simulink model "dspilbc"  (Simulink 8.3)
settings: Solver=FixedStepDiscrete  StartTime=0.0  StopTime=inf  RelTol=1e-3
InitFcn:
  | ilbcDatatype = get_param([bdroot '/Configuration'],'ilbcDialogDatatype');
  | if strcmp(get_param([bdroot '/Configuration'],'ilbcDialogMode'), '13.33 kbit/sec mode')
  |   ilbcMode = 1;
  | else
  |   ilbcMode = 2;
  | end
model workspace: external: MAT-File dspilbcdata.mat (data not in the file)
undefined symbols (not defined in the file or in its folder): dfilt, ilbc, Newton, Raphson
libraries: simulink x36, dspmtrx3 x27, dspsigops x13, dsparch4 x10, dspquant2 x9, dspilbclib x8, dspstat3 x8, dspsrcs4 x2, dspvision x1, dspmisc x1, dspsnks4 x1, dsplp x1
(part 1 of 3)
CloseFcn:
  | clear ilbcMode;
  | clear ilbcDatatype
settings Model: Creator=The MathWorks Inc.  ExtModeAutoUpdateStatusClock=off
settings DataIOCC: SaveOutput=off  SignalLogging=off  SaveTime=off
settings OptimizationCC: InlineParams=on  ExpressionDepthLimit=2147483647  InitFltsAndDblsToZero=on  EfficientFloat2IntCast=on  EfficientMapNaN2IntZero=off
settings DebuggingCC: InheritedTsInSrcMsg=none  SigSpecEnsureSampleTimeMsg=none  Int32ToFloatConvMsg=none  ParameterPrecisionLossMsg=none  FcnCallInpInsideContextMsg=UseLocalSettings  StrictBusMsg=ErrorOnBusTreatedAsVector
settings HardwareCC: ProdIntDivRoundTo=Floor
settings ModelReferenceCC: UpdateModelReferenceTargets=IfOutOfDate
settings SFSimCC: SimParseCustomCode=off
settings RTWCC: IncludeERTFirstTime=on
settings GRTTargetCC: TargetFcnLib=ansi_tfl_tmw_new.mat

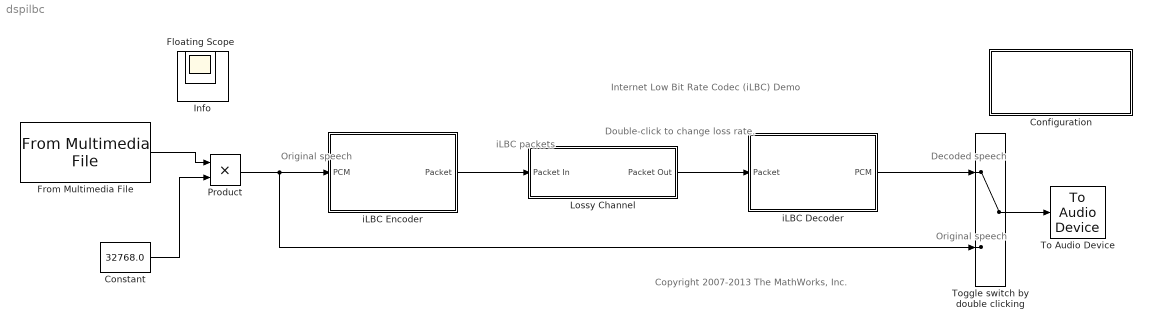
== system dspilbc ==
  note: Internet Low Bit Rate Codec (iLBC) Demo
  note: Original
      | speech
  note: iLBC
      | packets
  note: Double-click to change loss rate.
  note: Decoded
      | speech
  note: Original
      | speech
  note: Copyright 2007-2013 The MathWorks, Inc.
  Configuration : Subsystem  mask(iLBC Configuration){ilbcDialogMode=13.33 kbit/sec mode, ilbcDialogDatatype=double}
      mask prompts: ilbcDialogMode "iLBC mode:"; ilbcDialogDatatype "Internal data type:"
      mask help:
      | The iLBC standard is defined for two data rates: 13.33 kbit/sec and 15.20 kbit/sec.  Running under 13.33 kbit/sec, the encoder creates and outputs a compressed speech packet every 30ms.  With the 15.20 kbit/sec data rate, the encoder will output a packet every 20ms.  For the 13.33 kbit/sec mode, the packet size is a uint8 column vector of length 50, where each element represents one byte.  For the 15.20 kbit/sec mode, the packet is of length 38 bytes.
      |
      | The "Internal Data Type" option controls the precision for all internal floating point calculations in the iLBC Encoder and Decoder. The possible options are double and single precision.
      mask init:
      | if ilbcDialogMode == 1
      |     ilbcModeStr = '13.33';
      | elseif ilbcDialogMode == 2
      |     ilbcModeStr = '15.20';
      | end
      | 
      | if ilbcDialogDatatype == 1
      |     ilbcDatatype = 'double';
      | elseif ilbcDialogDatatype == 2
      |     ilbcDatatype = 'single';
      | end
      mask TypeOptions ilbcDialogMode: 13.33 kbit/sec mode | 15.20 kbit/sec mode
      mask TypeOptions ilbcDialogDatatype: double | single
      mask Display:
      | disp([ilbcModeStr ' kb/sec mode\n' ...
      |     'Internal data type: ' ilbcDatatype '\n' ...
      |     '[Double-click to change]']);
  Constant : Constant  Value=32768.0
  From Multimedia File : dspvision/From Multimedia File  inputFilename=speech_dft_8kHz.wav  loop=on  numPlays=inf  outputStreams=Audio only  videoDataType=single  audioDataType=double  inheritSampleTime=on  userDefinedSampleTime=1/30  noAudioOutput=off  isIntensityVideo=off  fourcc=RGB  colorVideoFormat=Separate color signals  outputEOF=off  dataOrg=Column-major  audioFrameSize=ilbc.BLOCKL{ilbcMode}  computeAudioFrameSize=off  outSamplingMode=Frame based
  Info : dspmisc/Info  SystemSampleTime=-1
  Lossy Channel : Subsystem  TreatAsAtomicUnit=on  mask(Lossy Channel){PercentLoss=3}
      mask prompts: PercentLoss "Percent of Packets Lost (0-100)"
      mask help:
      | This subsystem simulates a lossy channel by setting a specified percentage of packets to all zeros.  Enter the percentage of packets to be lost as a number in the range 0-100.
      |
      | Note that the packet loss concealment algorithm in the iLBC Decoder is tuned for packet loss rates between 0-10%.  Loss rates above 10% will result in decoded speech with clearly audible errors.
      mask Display: disp([num2str(PercentLoss) '% Random Packet Loss']);
  Product : Product  OutDataTypeStr=int16
  To Audio Device : dspsnks4/To Audio Device  deviceName=Default  inheritSampleRate=on  sampleRate=44100  deviceDatatype=Determine from input data type  autoBufferSize=on  bufferSize=4096  queueDuration=0.5  defaultOutputChannelMapping=on  outputChannelMapping=1
  Toggle switch by double clicking : ManualSwitch
  iLBC Decoder : Subsystem  TreatAsAtomicUnit=on
  iLBC Encoder : Subsystem  TreatAsAtomicUnit=on
  Floating Scope : Scope
      settings: Floating=on
  wires:
  iLBC Encoder/1(Packet) -> Lossy Channel/1(Packet In)
  Toggle switch by double clicking/1 -> To Audio Device/1
  Lossy Channel/1(Packet Out) -> iLBC Decoder/1(Packet)
  iLBC Decoder/1(PCM) -> Toggle switch by double clicking/1
  Constant/1 -> Product/2
  From Multimedia File/1 -> Product/1
  Product/1 -> Toggle switch by double clicking/2, iLBC Encoder/1(PCM)

== system dspilbc/Configuration ==

== system dspilbc/Lossy Channel ==
  Packet In : Inport
  Compare To Constant : simulink/Logic and Bit Operations/Compare To Constant  relop=>  const=PercentLoss  OutDataTypeStr=uint8  ZeroCross=off
  Gain : Gain  Gain=0  OutDataTypeStr=Inherit: Same as input
  Multiport Switch : MultiPortSwitch  DataPortOrder=Zero-based contiguous  Inputs=2  zeroidx=on
  Random Source : dspsrcs4/Random Source  SrcType=Uniform  NormMethod=Ziggurat  CltLength=12  MinVal=0  MaxVal=100  MeanVal=0  VarVal=1  RepMode=Not repeatable  rawSeed=1  IsInherit=off  SampMode=Discrete  SampTime=-1  SampFrame=1  DataType=Single  OutComplex=Real
  Packet Out : Outport
  wires:
  Multiport Switch/1 -> Packet Out/1
  Random Source/1 -> Compare To Constant/1
  Compare To Constant/1 -> Multiport Switch/1
  Packet In/1 -> Multiport Switch/3, Gain/1
  Gain/1 -> Multiport Switch/2

== system dspilbc/iLBC Decoder ==
  note: Section 4 of the iLBC standard
  Packet : Inport
  Data Type Duplicate : DataTypeDuplicate
  Data Type Duplicate1 : DataTypeDuplicate
  Data Type Conversion : DataTypeConversion  OutDataTypeStr=int16  SaturateOnIntegerOverflow=on
  Decode Sub-Blocks (4.1 - 4.4) : Subsystem
  Delay1 : dspsigops/Delay  InputProcessing=Columns as channels (frame based)  dly_unit=Frames  delay=1  ic_detail=off  dif_ic_for_ch=off  dif_ic_for_dly=off  ic=0  reset_popup=None
  Delay2 : dspsigops/Delay  InputProcessing=Columns as channels (frame based)  dly_unit=Frames  delay=1  ic_detail=off  dif_ic_for_ch=off  dif_ic_for_dly=off  ic=0  reset_popup=None
  Enable PLC : Constant  OutDataTypeStr=boolean
  High Pass Filter (4.8) : dsparch4/Digital Filter  TypePopup=IIR (poles & zeros)  IIRFiltStruct=Direct form II transposed  AllPoleFiltStruct=Direct form  FIRFiltStruct=Direct form  CoeffSource=Specify via dialog  NumCoeffs=ilbc.hpo_zero_coefsTbl  DenCoeffs=ilbc.hpo_pole_coefsTbl  BiQuadCoeffs=[1 0.3 0.4 1 0.1 0.2]  LatticeCoeffs=[0.2 0.4]  denIgnore=on  FiltPerSampPopup=One filter per frame  IC=0  ICnum=0  ICden=0  roundingMode=Floor  overflowMode=off  ScaleValues=1  scaleValueFracLength=14  stageInFracLength=15  stageOutFracLength=15  FilterSource=Specify via dialog  dfiltObjectName=dfilt.dffir([1 2 1])  InputProcessing=Columns as channels (frame based)
  Logical Operator : Logic  AllPortsSameDT=off  OutDataTypeStr=boolean
  Logical Operator1 : Logic  Operator=NOT  AllPortsSameDT=off  OutDataTypeStr=boolean
  Multiport Switch : MultiPortSwitch  DataPortOrder=Zero-based contiguous  Inputs=2  zeroidx=on
  Multiport Switch1 : MultiPortSwitch  DataPortOrder=Zero-based contiguous  Inputs=2  zeroidx=on
  Packet Loss Concealment (4.5) : Subsystem
  Saturation : Saturate  UpperLimit=32767  LowerLimit=-32768
  Set data type to back-propagate : Constant  OutDataTypeStr=ilbcDatatype
  Split Packet (3.8) : Subsystem  TreatAsAtomicUnit=on
  Synthesis Filtering (4.7) : Subsystem  TreatAsAtomicUnit=on
  PCM : Outport
  wires:
  Enable PLC/1 -> Logical Operator/2
  Set data type to back-propagate/1 -> Data Type Duplicate/1
  Logical Operator1/1 -> Logical Operator/1
  Logical Operator/1 -> Packet Loss Concealment (4.5)/Enable
  Packet Loss Concealment (4.5)/2(Synthesis) -> Multiport Switch1/2
  Packet Loss Concealment (4.5)/1(Residual) -> Multiport Switch/2
  Decode Sub-Blocks (4.1 - 4.4)/2(Synthesis) -> Data Type Duplicate1/2, Multiport Switch1/3
  Decode Sub-Blocks (4.1 - 4.4)/1(Residual) -> Multiport Switch/3
  Delay1/1 -> Packet Loss Concealment (4.5)/1(Last Residual)
  Delay2/1 -> Packet Loss Concealment (4.5)/2(Last Synthesis)
  Multiport Switch1/1 -> Data Type Duplicate1/1, Delay2/1, Synthesis Filtering (4.7)/2(Synthesis Filters)
  Multiport Switch/1 -> Delay1/1, Synthesis Filtering (4.7)/1(Residual)
  Split Packet (3.8)/8(Good Frame) -> Decode Sub-Blocks (4.1 - 4.4)/Enable, Multiport Switch1/1, Multiport Switch/1, Logical Operator1/1
  Split Packet (3.8)/1(Lsf Indices) -> Decode Sub-Blocks (4.1 - 4.4)/1(Lsf Indices)
  Split Packet (3.8)/7(Gain Indices) -> Decode Sub-Blocks (4.1 - 4.4)/7(Gain Indices)
  Split Packet (3.8)/6(Code Indices) -> Decode Sub-Blocks (4.1 - 4.4)/6(Code Indices)
  Split Packet (3.8)/5(Start State Indices) -> Decode Sub-Blocks (4.1 - 4.4)/5(Start State Indices)
  Split Packet (3.8)/4(Start State Gain Index) -> Decode Sub-Blocks (4.1 - 4.4)/4(Start State Gain Index)
  Split Packet (3.8)/3(State First) -> Decode Sub-Blocks (4.1 - 4.4)/3(State First)
  Split Packet (3.8)/2(Start State Number) -> Decode Sub-Blocks (4.1 - 4.4)/2(Start State Number)
  Synthesis Filtering (4.7)/1(Decoded Block) -> High Pass Filter (4.8)/1
  Saturation/1 -> Data Type Duplicate/2, Data Type Conversion/1
  Data Type Conversion/1 -> PCM/1
  Packet/1 -> Split Packet (3.8)/1(Packet)
  High Pass Filter (4.8)/1 -> Saturation/1

== system dspilbc/iLBC Encoder ==
  note: Section 3 of the iLBC standard
  PCM : Inport
  Calculate Residual (3.3) : Subsystem  TreatAsAtomicUnit=on
  Create Packet (3.8) : Subsystem  TreatAsAtomicUnit=on
  Data Type Conversion : DataTypeConversion  OutDataTypeStr=ilbcDatatype
  Encode Data (3.5 - 3.7) : Subsystem  TreatAsAtomicUnit=on
  Encoder LPC Analysis (3.2) : Subsystem  TreatAsAtomicUnit=on
  High Pass (3.1) : dsparch4/Digital Filter  TypePopup=IIR (poles & zeros)  IIRFiltStruct=Direct form II transposed  AllPoleFiltStruct=Direct form  FIRFiltStruct=Direct form  CoeffSource=Specify via dialog  NumCoeffs=ilbc.hpi_zero_coefsTbl  DenCoeffs=ilbc.hpi_pole_coefsTbl  BiQuadCoeffs=[1 0.3 0.4 1 0.1 0.2]  LatticeCoeffs=[0.2 0.4]  denIgnore=on  FiltPerSampPopup=One filter per frame  IC=0  ICnum=0  ICden=0  roundingMode=Floor  overflowMode=off  ScaleValues=1  scaleValueFracLength=14  stageInFracLength=15  stageOutFracLength=15  FilterSource=Specify via dialog  dfiltObjectName=dfilt.dffir([1 2 1])  InputProcessing=Columns as channels (frame based)
  Perceptual Weighting (3.4) : dspmtrx3/Array-Vector Multiply  mode=Mute  saveAsFlag=0  Dimension=1  V_Source=Dialog parameter  V_VectFromMask=ilbc.LPC_CHIRP_WEIGHTDENUM.^(0:10)'  firstCoeffSignedness=Auto  firstCoeffDataTypeStr=Inherit: Same word length as input  firstCoeffLastDataTypeStr=Inherit: Same word length as input  firstCoeffMin=[]  firstCoeffMax=[]  outputSignedness=Auto  outputDataTypeStr=Inherit: Same as product output  outputLastDataTypeStr=Inherit: Same as product output  outputMin=[]  outputMax=[]  accumSignedness=Auto  prodOutputSignedness=Auto  roundingMode=Floor  overflowMode=off
  Packet : Outport
  wires:
  Data Type Conversion/1 -> High Pass (3.1)/1
  Encoder LPC Analysis (3.2)/1(LSF Indices) -> Create Packet (3.8)/1(LSF Indices)
  High Pass (3.1)/1 -> Calculate Residual (3.3)/2(Data), Encoder LPC Analysis (3.2)/1(Data)
  Encode Data (3.5 - 3.7)/6(Gain Indices) -> Create Packet (3.8)/7(Gain Indices)
  Encode Data (3.5 - 3.7)/5(Code Indices) -> Create Packet (3.8)/6(Code Indices)
  Encode Data (3.5 - 3.7)/4(Start State Indices) -> Create Packet (3.8)/5(Start State Indices)
  Encode Data (3.5 - 3.7)/3(Start State Gain Index) -> Create Packet (3.8)/4(Start State Gain Index)
  Encode Data (3.5 - 3.7)/2(State First) -> Create Packet (3.8)/3(State First)
  Encode Data (3.5 - 3.7)/1(Start State Number) -> Create Packet (3.8)/2(Start State Number)
  Encoder LPC Analysis (3.2)/3(Weight Filters) -> Perceptual Weighting (3.4)/1
  Calculate Residual (3.3)/1(Residual) -> Encode Data (3.5 - 3.7)/3(Residual)
  Create Packet (3.8)/1(Packet) -> Packet/1
  PCM/1 -> Data Type Conversion/1
  Perceptual Weighting (3.4)/1 -> Encode Data (3.5 - 3.7)/2(Weights)
  Encoder LPC Analysis (3.2)/2(Synthesis Filters) -> Calculate Residual (3.3)/1(Synthesis Filters), Encode Data (3.5 - 3.7)/1(Synthesis)

== system dspilbc/iLBC Decoder/Decode Sub-Blocks (4.1 - 4.4) ==
  Lsf Indices : Inport
  Start State Number : Inport  Port=2
  State First : Inport  Port=3
  Start State Gain Index : Inport  Port=4
  Start State Indices : Inport  Port=5
  Code Indices : Inport  Port=6
  Gain Indices : Inport  Port=7
  Enable : EnablePort
  Decode Remaining Sub-Blocks (4.3 - 4.4) : Subsystem  TreatAsAtomicUnit=on
  Decode Start State : dspilbclib/Decode Start State
  Decoder LPC Analysis (4.1) : Subsystem  TreatAsAtomicUnit=on
  Frame Conversion2 : FrameConversion  OutFrame=Sample-based
  Selector1 : Selector  NumberOfDimensions=2  InputPortWidth=3  IndexOptions=Select all,Index vector (port)  Indices=-1,-1
  Residual : Outport
  Synthesis : Outport  Port=2
  wires:
  Frame Conversion2/1 -> Decode Remaining Sub-Blocks (4.3 - 4.4)/1(Initial Codebook)
  Start State Number/1 -> Selector1/2, Decode Remaining Sub-Blocks (4.3 - 4.4)/4(Start State Number)
  Selector1/1 -> Decode Start State/3
  State First/1 -> Decode Start State/4, Decode Remaining Sub-Blocks (4.3 - 4.4)/5(State First)
  Lsf Indices/1 -> Decoder LPC Analysis (4.1)/1(LSF Indices)
  Decoder LPC Analysis (4.1)/1(Synthesis) -> Synthesis/1, Selector1/1
  Start State Indices/1 -> Decode Start State/1
  Start State Gain Index/1 -> Decode Start State/2
  Decode Start State/1 -> Frame Conversion2/1
  Code Indices/1 -> Decode Remaining Sub-Blocks (4.3 - 4.4)/2(Code Indices)
  Gain Indices/1 -> Decode Remaining Sub-Blocks (4.3 - 4.4)/3(Gain Indices)
  Decode Remaining Sub-Blocks (4.3 - 4.4)/1(Residual) -> Residual/1

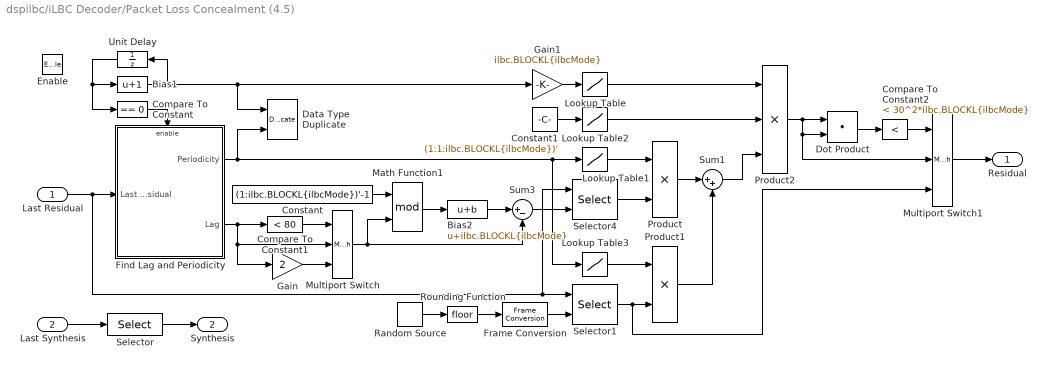
== system dspilbc/iLBC Decoder/Packet Loss Concealment (4.5) ==
  Last Residual : Inport
  Last Synthesis : Inport  Port=2
  Enable : EnablePort  StatesWhenEnabling=reset
  Bias1 : Bias  Bias=1
  Bias2 : Bias  Bias=ilbc.BLOCKL{ilbcMode}
  Compare To Constant : simulink/Logic and Bit Operations/Compare To Constant  relop===  const=0  OutDataTypeStr=boolean  ZeroCross=off
  Compare To Constant1 : simulink/Logic and Bit Operations/Compare To Constant  relop=<  const=80  OutDataTypeStr=uint8  ZeroCross=off
  Compare To Constant2 : simulink/Logic and Bit Operations/Compare To Constant  relop=<  const=30^2*ilbc.BLOCKL{ilbcMode}  OutDataTypeStr=boolean  ZeroCross=off
  Constant : Constant  Value=(1:ilbc.BLOCKL{ilbcMode})'-1  VectorParams1D=off  OutDataTypeStr=Inherit: Inherit via back propagation
  Constant1 : Constant  Value=(1:1:ilbc.BLOCKL{ilbcMode})'  VectorParams1D=off  OutDataTypeStr=Inherit: Inherit via back propagation
  Data Type Duplicate : DataTypeDuplicate
  Dot Product : DotProduct  InputSameDT=on  OutDataTypeStr=Inherit: Inherit via internal rule
  Find Lag and Periodicity : Subsystem  TreatAsAtomicUnit=on
  Frame Conversion : FrameConversion  OutFrame=Sample-based
  Gain : Gain  Gain=2  OutDataTypeStr=Inherit: Same as input
  Gain1 : Gain  Gain=ilbc.BLOCKL{ilbcMode}  OutDataTypeStr=Inherit: Inherit via back propagation  ParamDataTypeStr=Inherit: Same as input
  Lookup Table : Lookup_n-D  NumberOfTableDimensions=1  BreakpointsForDimension1=[0 320 640 960 1280]  Table=[1.0 0.9 0.7 0.5 0.0]  InterpMethod=Flat  InputSameDT=on
  Lookup Table1 : Lookup_n-D  NumberOfTableDimensions=1  BreakpointsForDimension1=[0.3 0.6]  Table=[0 1]  ExtrapMethod=Clip  InputSameDT=on
  Lookup Table2 : Lookup_n-D  NumberOfTableDimensions=1  BreakpointsForDimension1=[80 160 240]  Table=[1.00 0.95 0.90]  ExtrapMethod=Clip  InputSameDT=on
  Lookup Table3 : Lookup_n-D  NumberOfTableDimensions=1  BreakpointsForDimension1=[0.3 0.6]  Table=[1 0]  ExtrapMethod=Clip  InputSameDT=on
  Math Function1 : Math  Operator=mod  SaturateOnIntegerOverflow=on
  Multiport Switch : MultiPortSwitch  DataPortOrder=Zero-based contiguous  Inputs=2  zeroidx=on
  Multiport Switch1 : MultiPortSwitch  DataPortOrder=Zero-based contiguous  Inputs=2  zeroidx=on
  Product : Product  RndMeth=Zero
  Product1 : Product  RndMeth=Zero
  Product2 : Product  Inputs=3  RndMeth=Zero  OutDataTypeStr=Inherit: Same as first input
  Random Source : dspsrcs4/Random Source  SrcType=Uniform  NormMethod=Ziggurat  CltLength=12  MinVal=ilbc.BLOCKL{ilbcMode}-70  MaxVal=ilbc.BLOCKL{ilbcMode}-0.001  MeanVal=0  VarVal=1  RepMode=Not repeatable  rawSeed=1  IsInherit=off  SampMode=Discrete  SampTime=-1  SampFrame=ilbc.BLOCKL{ilbcMode}  DataType=Single  OutComplex=Real
  Rounding Function : Rounding
  Selector : Selector  NumberOfDimensions=2  InputPortWidth=3  IndexOptions=Select all,Index vector (dialog)  Indices=[1 3],repmat(ilbc.NSUB{ilbcMode},1,ilbc.NSUB{ilbcMode})  OutputSizes=1,1
  Selector1 : Selector  NumberOfDimensions=2  IndexMode=Zero-based  InputPortWidth=3  IndexOptions=Index vector (port),Select all  Indices=[1 3],1  OutputSizes=1,1
  Selector4 : Selector  NumberOfDimensions=2  IndexMode=Zero-based  InputPortWidth=3  IndexOptions=Index vector (port),Select all  Indices=[1 3],1  OutputSizes=1,1
  Sum1 : Sum  Inputs=|++
  Sum3 : Sum  Inputs=|+-
  Unit Delay : UnitDelay  SampleTime=-1
  Residual : Outport
  Synthesis : Outport  Port=2
  wires:
  Bias1/1 -> Data Type Duplicate/1, Gain1/1, Unit Delay/1
  Frame Conversion/1 -> Selector1/2
  Unit Delay/1 -> Compare To Constant/1, Bias1/1
  Compare To Constant/1 -> Find Lag and Periodicity/Enable
  Random Source/1 -> Rounding Function/1
  Rounding Function/1 -> Frame Conversion/1
  Gain/1 -> Multiport Switch/3
  Product1/1 -> Sum1/2
  Product/1 -> Sum1/1
  Selector1/1 -> Multiport Switch1/3, Product1/2
  Lookup Table3/1 -> Product1/1
  Selector4/1 -> Product/2
  Lookup Table1/1 -> Product/1
  Multiport Switch/1 -> Sum3/2, Math Function1/2
  Sum3/1 -> Selector4/2
  Bias2/1 -> Sum3/1
  Math Function1/1 -> Bias2/1
  Constant/1 -> Math Function1/1
  Product2/1 -> Multiport Switch1/2, Dot Product/2, Dot Product/1
  Last Residual/1 -> Selector1/1, Selector4/1, Find Lag and Periodicity/1(Last Residual)
  Lookup Table2/1 -> Product2/2
  Lookup Table/1 -> Product2/1
  Multiport Switch1/1 -> Residual/1
  Compare To Constant2/1 -> Multiport Switch1/1
  Dot Product/1 -> Compare To Constant2/1
  Sum1/1 -> Product2/3
  Constant1/1 -> Lookup Table2/1
  Gain1/1 -> Lookup Table/1
  Compare To Constant1/1 -> Multiport Switch/1
  Find Lag and Periodicity/1(Periodicity) -> Data Type Duplicate/2, Lookup Table3/1, Lookup Table1/1
  Find Lag and Periodicity/2(Lag) -> Gain/1, Multiport Switch/2, Compare To Constant1/1
  Selector/1 -> Synthesis/1
  Last Synthesis/1 -> Selector/1

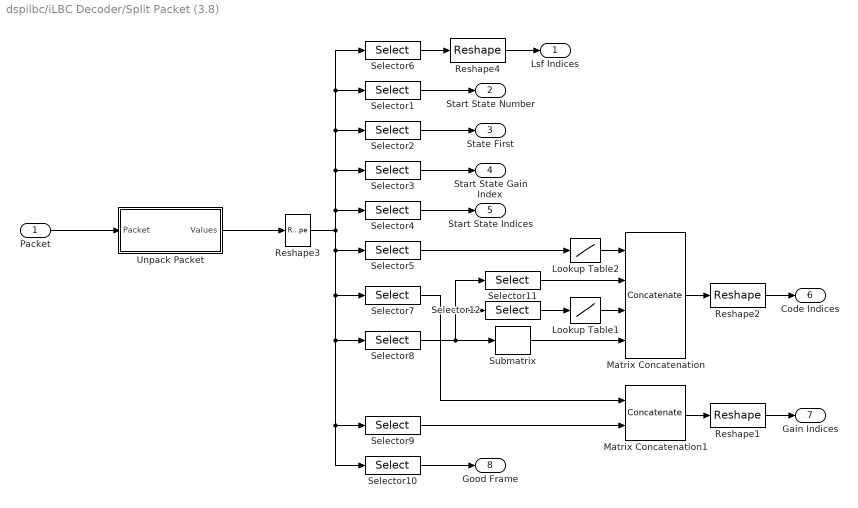
== system dspilbc/iLBC Decoder/Split Packet (3.8) ==
  Packet : Inport
  Lookup Table1 : Lookup_n-D  NumberOfTableDimensions=1  BreakpointsForDimension1=[0:255]  Table=[0:43 108:171 236:255 zeros(1,128)]  ExtrapMethod=Clip  InputSameDT=on
  Lookup Table2 : Lookup_n-D  NumberOfTableDimensions=1  BreakpointsForDimension1=[0:255]  Table=[0:57 zeros(1,6) 128:185 zeros(1,134)]  ExtrapMethod=Clip  InputSameDT=on
  Matrix Concatenation : Concatenate  NumInputs=4  Mode=Multidimensional array
  Matrix Concatenation1 : Concatenate  Mode=Multidimensional array
  Reshape1 : Reshape  OutputDimensionality=Customize  OutputDimensions=[3 (ilbc.NSUB{ilbcMode}-1)]
  Reshape2 : Reshape  OutputDimensionality=Customize  OutputDimensions=[3 (ilbc.NSUB{ilbcMode}-1)]
  Reshape3 : Reshape  OutputDimensionality=Column vector (2-D)
  Reshape4 : Reshape  OutputDimensionality=Customize  OutputDimensions=[3 (3-ilbcMode)]
  Selector1 : Selector  NumberOfDimensions=2  InputPortWidth=3  IndexOptions=Index vector (dialog),Select all  Indices=ilbc.packet_idxTbl{ilbcMode}{2},-1
  Selector10 : Selector  NumberOfDimensions=2  InputPortWidth=3  IndexOptions=Index vector (dialog),Select all  Indices=ilbc.packet_idxTbl{ilbcMode}{10},-1
  Selector11 : Selector  NumberOfDimensions=2  InputPortWidth=3  IndexOptions=Index vector (dialog),Select all  Indices=1,-1
  Selector12 : Selector  NumberOfDimensions=2  InputPortWidth=3  IndexOptions=Index vector (dialog),Select all  Indices=2:3,-1
  Selector2 : Selector  NumberOfDimensions=2  InputPortWidth=3  IndexOptions=Index vector (dialog),Select all  Indices=ilbc.packet_idxTbl{ilbcMode}{3},-1
  Selector3 : Selector  NumberOfDimensions=2  InputPortWidth=3  IndexOptions=Index vector (dialog),Select all  Indices=ilbc.packet_idxTbl{ilbcMode}{4},-1
  Selector4 : Selector  NumberOfDimensions=2  InputPortWidth=3  IndexOptions=Index vector (dialog),Select all  Indices=ilbc.packet_idxTbl{ilbcMode}{5},-1
  Selector5 : Selector  NumberOfDimensions=2  InputPortWidth=3  IndexOptions=Index vector (dialog),Select all  Indices=ilbc.packet_idxTbl{ilbcMode}{6},-1
  Selector6 : Selector  NumberOfDimensions=2  InputPortWidth=3  IndexOptions=Index vector (dialog),Select all  Indices=ilbc.packet_idxTbl{ilbcMode}{1},-1
  Selector7 : Selector  NumberOfDimensions=2  InputPortWidth=3  IndexOptions=Index vector (dialog),Select all  Indices=ilbc.packet_idxTbl{ilbcMode}{7},-1
  Selector8 : Selector  NumberOfDimensions=2  InputPortWidth=3  IndexOptions=Index vector (dialog),Select all  Indices=ilbc.packet_idxTbl{ilbcMode}{8},-1
  Selector9 : Selector  NumberOfDimensions=2  InputPortWidth=3  IndexOptions=Index vector (dialog),Select all  Indices=ilbc.packet_idxTbl{ilbcMode}{9},-1
  Submatrix : dspmtrx3/Submatrix  RowSpan=Range of rows  RowStartMode=Index  RowStartIndex=4  RowEndMode=Last  RowEndIndex=1  ColSpan=All columns  ColStartMode=First  ColStartIndex=1  ColEndMode=Last  ColEndIndex=1
  Unpack Packet : Subsystem  TreatAsAtomicUnit=on
  Lsf Indices : Outport
  Start State Number : Outport  Port=2
  State First : Outport  Port=3
  Start State Gain Index : Outport  Port=4
  Start State Indices : Outport  Port=5
  Code Indices : Outport  Port=6
  Gain Indices : Outport  Port=7
  Good Frame : Outport  Port=8
  wires:
  Unpack Packet/1(Values) -> Reshape3/1
  Packet/1 -> Unpack Packet/1(Packet)
  Lookup Table1/1 -> Matrix Concatenation/3
  Lookup Table2/1 -> Matrix Concatenation/1
  Selector12/1 -> Lookup Table1/1
  Selector11/1 -> Matrix Concatenation/2
  Submatrix/1 -> Matrix Concatenation/4
  Selector8/1 -> Submatrix/1, Selector12/1, Selector11/1
  Selector5/1 -> Lookup Table2/1
  Reshape4/1 -> Lsf Indices/1
  Reshape3/1 -> Selector1/1, Selector6/1, Selector2/1, Selector3/1, Selector4/1, Selector5/1, Selector7/1, Selector9/1, Selector10/1, Selector8/1
  Selector6/1 -> Reshape4/1
  Selector10/1 -> Good Frame/1
  Selector7/1 -> Matrix Concatenation1/1
  Selector9/1 -> Matrix Concatenation1/2
  Selector2/1 -> State First/1
  Selector4/1 -> Start State Indices/1
  Selector3/1 -> Start State Gain Index/1
  Selector1/1 -> Start State Number/1
  Reshape1/1 -> Gain Indices/1
  Reshape2/1 -> Code Indices/1
  Matrix Concatenation1/1 -> Reshape1/1
  Matrix Concatenation/1 -> Reshape2/1

== system dspilbc/iLBC Decoder/Synthesis Filtering (4.7) ==
  Residual : Inport
  Synthesis Filters : Inport  Port=2
  Assignment : Assignment  NumberOfDimensions=2  OutputInitialize=Specify size for each dimension in table  IndexOptions=Assign all,Index vector (port)  Indices=-1,1  OutputSizes=40,ilbc.NSUB{ilbcMode}
  For Iterator : ForIterator  IterationLimit=ilbc.NSUB{ilbcMode}  IterationVariableDataType=int8
  Reshape : Reshape  OutputDimensionality=Customize  OutputDimensions=[40 ilbc.NSUB{ilbcMode}]
  Reshape1 : Reshape  OutputDimensionality=Column vector (2-D)  OutputDimensions=[50 4]
  Selector1 : Selector  NumberOfDimensions=2  InputPortWidth=3  IndexOptions=Select all,Index vector (port)  Indices=-1,-1
  Selector2 : Selector  NumberOfDimensions=2  InputPortWidth=3  IndexOptions=Select all,Index vector (port)  Indices=-1,-1
  Time-Varying  Analysis Filter3 : dsparch4/Digital Filter  TypePopup=IIR (all poles)  IIRFiltStruct=Direct form II transposed  AllPoleFiltStruct=Direct form  FIRFiltStruct=Direct form  CoeffSource=Input port(s)  NumCoeffs=[1 -.95]  DenCoeffs=[1 0.1]  BiQuadCoeffs=[1 0.3 0.4 1 0.1 0.2]  LatticeCoeffs=[0.2 0.4]  denIgnore=on  FiltPerSampPopup=One filter per frame  IC=0  ICnum=0  ICden=0  roundingMode=Floor  overflowMode=off  ScaleValues=1  scaleValueFracLength=14  stageInFracLength=15  stageOutFracLength=15  FilterSource=Input port(s)  dfiltObjectName=dfilt.dffir([1 2 1])  InputProcessing=Columns as channels (frame based)
  Decoded Block : Outport
  wires:
  Reshape1/1 -> Decoded Block/1
  Assignment/1 -> Reshape1/1
  Selector1/1 -> Time-Varying  Analysis Filter3/2
  Time-Varying  Analysis Filter3/1 -> Assignment/1
  Reshape/1 -> Selector2/1
  For Iterator/1 -> Assignment/2, Selector2/2, Selector1/2
  Selector2/1 -> Time-Varying  Analysis Filter3/1
  Synthesis Filters/1 -> Selector1/1
  Residual/1 -> Reshape/1

== system dspilbc/iLBC Encoder/Calculate Residual (3.3) ==
  Synthesis Filters : Inport
  Data : Inport  Port=2
  Assignment1 : Assignment  NumberOfDimensions=2  OutputInitialize=Specify size for each dimension in table  IndexOptions=Assign all,Index vector (port)  Indices=-1,1  OutputSizes=40,ilbc.NSUB{ilbcMode}
  For Iterator : ForIterator  IterationLimit=ilbc.NSUB{ilbcMode}  IterationVariableDataType=int8
  Reshape2 : Reshape  OutputDimensionality=Customize  OutputDimensions=[40 ilbc.NSUB{ilbcMode}]
  Selector1 : Selector  NumberOfDimensions=2  InputPortWidth=3  IndexOptions=Select all,Index vector (port)  Indices=-1,-1
  Selector2 : Selector  NumberOfDimensions=2  InputPortWidth=3  IndexOptions=Select all,Index vector (port)  Indices=-1,-1
  Time-Varying  Analysis Filter1 : dsparch4/Digital Filter  TypePopup=FIR (all zeros)  IIRFiltStruct=Direct form II transposed  AllPoleFiltStruct=Direct form  FIRFiltStruct=Direct form  CoeffSource=Input port(s)  NumCoeffs=[1 -.95]  DenCoeffs=[1 0.1]  BiQuadCoeffs=[1 0.3 0.4 1 0.1 0.2]  LatticeCoeffs=[0.2 0.4]  denIgnore=on  FiltPerSampPopup=One filter per frame  IC=0  ICnum=0  ICden=0  roundingMode=Floor  overflowMode=off  ScaleValues=1  scaleValueFracLength=14  stageInFracLength=15  stageOutFracLength=15  FilterSource=Input port(s)  dfiltObjectName=dfilt.dffir([1 2 1])  InputProcessing=Columns as channels (frame based)
  Residual : Outport
  wires:
  Time-Varying  Analysis Filter1/1 -> Assignment1/1
  Selector1/1 -> Time-Varying  Analysis Filter1/2
  Selector2/1 -> Time-Varying  Analysis Filter1/1
  Assignment1/1 -> Residual/1
  Synthesis Filters/1 -> Selector1/1
  Data/1 -> Reshape2/1
  Reshape2/1 -> Selector2/1
  For Iterator/1 -> Selector1/2, Selector2/2, Assignment1/2

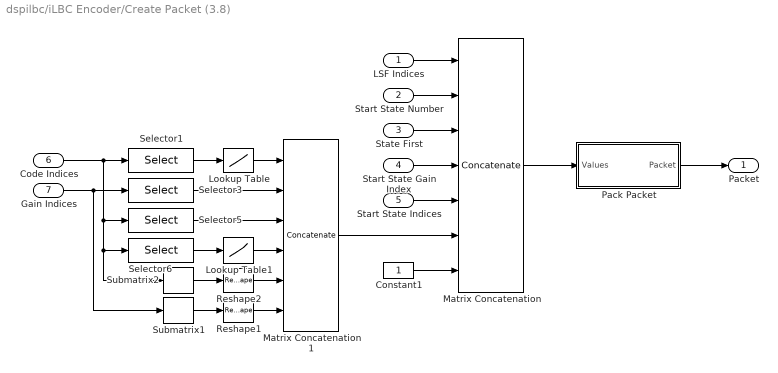
== system dspilbc/iLBC Encoder/Create Packet (3.8) ==
  LSF Indices : Inport
  Start State Number : Inport  Port=2
  State First : Inport  Port=3
  Start State Gain Index : Inport  Port=4
  Start State Indices : Inport  Port=5
  Code Indices : Inport  Port=6
  Gain Indices : Inport  Port=7
  Constant1 : Constant  OutDataTypeStr=uint8
  Lookup Table : Lookup_n-D  NumberOfTableDimensions=1  BreakpointsForDimension1=[0:255]  Table=[0:57 zeros(1,70) 64:121 zeros(1,70)]  ExtrapMethod=Clip  InputSameDT=on
  Lookup Table1 : Lookup_n-D  NumberOfTableDimensions=1  BreakpointsForDimension1=[0:255]  Table=[0:43 zeros(1,64) 44:107 zeros(1,64) 108:127]  ExtrapMethod=Clip  InputSameDT=on
  Matrix Concatenation : Concatenate  NumInputs=7  Mode=Multidimensional array
  Matrix Concatenation1 : Concatenate  NumInputs=6  Mode=Multidimensional array
  Pack Packet : Subsystem  TreatAsAtomicUnit=on
  Reshape1 : Reshape  OutputDimensionality=Column vector (2-D)
  Reshape2 : Reshape  OutputDimensionality=Column vector (2-D)
  Selector1 : Selector  NumberOfDimensions=2  InputPortWidth=3  IndexOptions=Select all,Index vector (dialog)  Indices=-1,1
  Selector3 : Selector  NumberOfDimensions=2  InputPortWidth=3  IndexOptions=Select all,Index vector (dialog)  Indices=-1,1
  Selector5 : Selector  NumberOfDimensions=2  InputPortWidth=3  IndexOptions=Index vector (dialog),Index vector (dialog)  Indices=1,2
  Selector6 : Selector  NumberOfDimensions=2  InputPortWidth=3  IndexOptions=Index vector (dialog),Index vector (dialog)  Indices=2:3,2
  Submatrix1 : dspmtrx3/Submatrix  RowSpan=All rows  RowStartMode=First  RowStartIndex=1  RowEndMode=Last  RowEndIndex=1  ColSpan=Range of columns  ColStartMode=Index  ColStartIndex=2  ColEndMode=Last  ColEndIndex=1
  Submatrix2 : dspmtrx3/Submatrix  RowSpan=All rows  RowStartMode=First  RowStartIndex=1  RowEndMode=Last  RowEndIndex=1  ColSpan=Range of columns  ColStartMode=Index  ColStartIndex=3  ColEndMode=Last  ColEndIndex=1
  Packet : Outport
  wires:
  Pack Packet/1(Packet) -> Packet/1
  Matrix Concatenation/1 -> Pack Packet/1(Values)
  Lookup Table1/1 -> Matrix Concatenation1/4
  Lookup Table/1 -> Matrix Concatenation1/1
  Selector3/1 -> Matrix Concatenation1/2
  Gain Indices/1 -> Submatrix1/1, Selector3/1
  Reshape1/1 -> Matrix Concatenation1/6
  Reshape2/1 -> Matrix Concatenation1/5
  Submatrix2/1 -> Reshape2/1
  Selector5/1 -> Matrix Concatenation1/3
  Selector6/1 -> Lookup Table1/1
  Submatrix1/1 -> Reshape1/1
  Matrix Concatenation1/1 -> Matrix Concatenation/6
  Selector1/1 -> Lookup Table/1
  Code Indices/1 -> Submatrix2/1, Selector6/1, Selector5/1, Selector1/1
  Constant1/1 -> Matrix Concatenation/7
  Start State Indices/1 -> Matrix Concatenation/5
  Start State Gain Index/1 -> Matrix Concatenation/4
  State First/1 -> Matrix Concatenation/3
  Start State Number/1 -> Matrix Concatenation/2
  LSF Indices/1 -> Matrix Concatenation/1

== system dspilbc/iLBC Encoder/Encode Data (3.5 - 3.7) ==
  Synthesis : Inport
  Weights : Inport  Port=2
  Residual : Inport  Port=3
  Decode Start State (3.5.3 last paragraph) : dspilbclib/Decode Start State
  Encode Remaining Sub-Blocks (3.6 - 3.7) : Subsystem
  Encode Start State (3.5.2 - 3.5.3) : Subsystem  TreatAsAtomicUnit=on
  Extract Sub-Blocks (3.5.1) and Sort LPC Filters : Subsystem  TreatAsAtomicUnit=on
  Start State Number : Outport
  State First : Outport  Port=2
  Start State Gain Index : Outport  Port=3
  Start State Indices : Outport  Port=4
  Code Indices : Outport  Port=5
  Gain Indices : Outport  Port=6
  wires:
  Extract Sub-Blocks (3.5.1) and Sort LPC Filters/3(Start State Number) -> Start State Number/1, Encode Remaining Sub-Blocks (3.6 - 3.7)/3(Start State Number)
  Extract Sub-Blocks (3.5.1) and Sort LPC Filters/7(Start State Synthesis) -> Decode Start State (3.5.3 last paragraph)/3, Encode Start State (3.5.2 - 3.5.3)/3(Synthesis Filter)
  Extract Sub-Blocks (3.5.1) and Sort LPC Filters/6(Start State Weights) -> Encode Start State (3.5.2 - 3.5.3)/2(Weight Filters)
  Extract Sub-Blocks (3.5.1) and Sort LPC Filters/5(Start State) -> Encode Start State (3.5.2 - 3.5.3)/1(Start State)
  Weights/1 -> Extract Sub-Blocks (3.5.1) and Sort LPC Filters/3(Weights)
  Extract Sub-Blocks (3.5.1) and Sort LPC Filters/2(Sorted Weights) -> Encode Remaining Sub-Blocks (3.6 - 3.7)/2(Weights)
  Extract Sub-Blocks (3.5.1) and Sort LPC Filters/1(Sorted Sub-blocks) -> Encode Remaining Sub-Blocks (3.6 - 3.7)/1(Sub-blocks)
  Synthesis/1 -> Extract Sub-Blocks (3.5.1) and Sort LPC Filters/2(Synthesis)
  Encode Start State (3.5.2 - 3.5.3)/2(Start State Gain Index) -> Start State Gain Index/1, Decode Start State (3.5.3 last paragraph)/2
  Decode Start State (3.5.3 last paragraph)/1 -> Encode Remaining Sub-Blocks (3.6 - 3.7)/5(Initial Codebook)
  Encode Remaining Sub-Blocks (3.6 - 3.7)/2(Gains) -> Gain Indices/1
  Encode Remaining Sub-Blocks (3.6 - 3.7)/1(Codes) -> Code Indices/1
  Encode Start State (3.5.2 - 3.5.3)/1(Start State Indices) -> Start State Indices/1, Decode Start State (3.5.3 last paragraph)/1
  Residual/1 -> Extract Sub-Blocks (3.5.1) and Sort LPC Filters/1(Residual)
  Extract Sub-Blocks (3.5.1) and Sort LPC Filters/4(State First) -> Encode Remaining Sub-Blocks (3.6 - 3.7)/4(State First), State First/1, Decode Start State (3.5.3 last paragraph)/4, Encode Start State (3.5.2 - 3.5.3)/4(State First)

== system dspilbc/iLBC Encoder/Encoder LPC Analysis (3.2) ==
  note: 3.2.1
  note: 3.2.2
  note: 3.2.3
  Data : Inport
  Autocorrelation : dspstat3/Autocorrelation  AllPositiveLags=off  maxlag=10  bias=None  domain=Time  outputDataTypeStr=Inherit: Same as accumulator  outputLastDataTypeStr=Inherit: Same as accumulator  outputMin=[]  outputMax=[]  roundingMode=Floor  overflowMode=off
  Delay2 : dspsigops/Delay  InputProcessing=Columns as channels (frame based)  dly_unit=Frames  delay=1  ic_detail=off  dif_ic_for_ch=off  dif_ic_for_dly=off  ic=0  reset_popup=None
  Find Perceptual Weight Filters (3.2.6) : dspilbclib/Find LPC Filters
  Find Synthesis Filters (3.2.6) : dspilbclib/Find LPC Filters
  Frame Conversion1 : FrameConversion
  Gain : Gain  Gain=ilbc.lpc_winTbls{ilbcMode}
  LPC to LSF/LSP Conversion1 : dsplp/LPC to LSF//LSP Conversion  output=LSF in range (0 pi)  NSteps=64  NBisects=6  RootStatus=off  correction=off  lastLSP=off  error=Ignore
  LSF Quantization (3.2.4) : Subsystem
  Levinson-Durbin : dspsolvers/Levinson-Durbin  coeffOutFcn=OBSOLETE  coeffOutFcnActive=A  outP=off  zeroInpHandling=on  firstCoeffMode=Binary point scaling  firstCoeffWordLength=16  firstCoeffFracLength=15  firstCoeffDataTypeStr=fixdt(1,16,15)  firstCoeffLastDataTypeStr=fixdt(1,16,15)  firstCoeffMin=[]  firstCoeffMax=[]  secondCoeffMode=Binary point scaling  secondCoeffWordLength=16  secondCoeffFracLength=15  secondCoeffDataTypeStr=fixdt(1,16,15)  secondCoeffLastDataTypeStr=fixdt(1,16,15)  secondCoeffMin=[]  secondCoeffMax=[]  outputMin=[]  outputMax=[]  accumMode=Binary point scaling  accumWordLength=32  accumFracLength=30  accumDataTypeStr=fixdt(1,32,30)  accumLastDataTypeStr=fixdt(1,32,30)  prodOutputMode=Binary point scaling  prodOutputWordLength=32  prodOutputFracLength=30  prodOutputDataTypeStr=fixdt(1,32,30)  prodOutputLastDataTypeStr=fixdt(1,32,30)  roundingMode=Floor  overflowMode=off
      settings: allowOverrides=off
  Matrix Concatenation3 : Concatenate  Mode=Multidimensional array
  Matrix Scaling : dspmtrx3/Array-Vector Multiply  mode=Mute  saveAsFlag=0  Dimension=1  V_Source=Dialog parameter  V_VectFromMask=ilbc.lpc_lagwinTbl  firstCoeffSignedness=Auto  firstCoeffDataTypeStr=Inherit: Same word length as input  firstCoeffLastDataTypeStr=Inherit: Same word length as input  firstCoeffMin=[]  firstCoeffMax=[]  outputSignedness=Auto  outputDataTypeStr=Inherit: Same as product output  outputLastDataTypeStr=Inherit: Same as product output  outputMin=[]  outputMax=[]  accumSignedness=Auto  prodOutputSignedness=Auto  roundingMode=Floor  overflowMode=off
  Matrix Scaling1 : dspmtrx3/Array-Vector Multiply  mode=Mute  saveAsFlag=0  Dimension=1  V_Source=Dialog parameter  V_VectFromMask=ilbc.LPC_CHIRP_SYNTDENUM.^(0:10)'  firstCoeffSignedness=Auto  firstCoeffDataTypeStr=Inherit: Same word length as input  firstCoeffLastDataTypeStr=Inherit: Same word length as input  firstCoeffMin=[]  firstCoeffMax=[]  outputSignedness=Auto  outputDataTypeStr=Inherit: Same as product output  outputLastDataTypeStr=Inherit: Same as product output  outputMin=[]  outputMax=[]  accumSignedness=Auto  prodOutputSignedness=Auto  roundingMode=Floor  overflowMode=off
  Reshape : Reshape  OutputDimensionality=Customize  OutputDimensions=[240 (3-ilbcMode)]
  Selector : Selector  NumberOfDimensions=2  InputPortWidth=3  IndexOptions=Index vector (dialog),Index vector (dialog)  Indices=ilbc.lpc_winIdxTbl{ilbcMode},1  OutputSizes=1,1
  Submatrix1 : dspmtrx3/Submatrix  RowSpan=Range of rows  RowStartMode=Offset from last  RowStartIndex=ilbc.BUFFEROVERLAP{ilbcMode}-1  RowEndMode=Last  RowEndIndex=1  ColSpan=All columns  ColStartMode=Offset from last  ColStartIndex=1  ColEndMode=Last  ColEndIndex=1
  LSF Indices : Outport
  Synthesis Filters : Outport  Port=2
  Weight Filters : Outport  Port=3
  wires:
  Matrix Concatenation3/1 -> Selector/1
  Data/1 -> Matrix Concatenation3/2, Submatrix1/1
  Submatrix1/1 -> Delay2/1
  Delay2/1 -> Matrix Concatenation3/1
  Selector/1 -> Reshape/1
  Autocorrelation/1 -> Matrix Scaling/1
  LSF Quantization (3.2.4)/2(Quantized LSF Vectors) -> Find Synthesis Filters (3.2.6)/1
  Gain/1 -> Autocorrelation/1
  LSF Quantization (3.2.4)/1(LSF Indices) -> LSF Indices/1
  Reshape/1 -> Gain/1
  Levinson-Durbin/1 -> Matrix Scaling1/1
  Matrix Scaling1/1 -> LPC to LSF/LSP Conversion1/1
  Find Synthesis Filters (3.2.6)/1 -> Synthesis Filters/1
  Find Perceptual Weight Filters (3.2.6)/1 -> Weight Filters/1
  Frame Conversion1/1 -> LSF Quantization (3.2.4)/1(LSF Vectors), Find Perceptual Weight Filters (3.2.6)/1
  LPC to LSF/LSP Conversion1/1 -> Frame Conversion1/1
  Matrix Scaling/1 -> Levinson-Durbin/1

== system dspilbc/iLBC Decoder/Decode Sub-Blocks (4.1 - 4.4)/Decode Remaining Sub-Blocks (4.3 - 4.4) ==
  Initial Codebook : Inport
  Code Indices : Inport  Port=2
  Gain Indices : Inport  Port=3
  Start State Number : Inport  Port=4
  State First : Inport  Port=5
  Compare To Constant2 : simulink/Logic and Bit Operations/Compare To Constant  relop=>  const=0  OutDataTypeStr=uint8  ZeroCross=off
  Decode Remaining Sub-Blocks (4.3 - 4.4) : dspilbclib/Decode Sub-Block
  For Iterator : ForIterator  ResetStates=reset  IterationLimit=ilbc.NSUB{ilbcMode}-1  IndexMode=Zero-based
  Frame Conversion1 : FrameConversion  OutFrame=Sample-based
  Frame Conversion3 : FrameConversion
  Pad : dspsigops/Pad  padAlong=Columns  dimsToPad=1  valSrc=Specify via dialog  padVal=0  spec=Pad size  padNumOutRowsSpecMethod=User-specified  numOutRows=ilbc.BLOCKL{ilbcMode}-40  padNumOutColsSpecMethod=User-specified  numOutCols=1  isVarDimsMode=off  padBeginning=90  padEnd=0  outSizeMode=User-specified  outSize=1  padSigAt=Beginning  trunc_flag=None  roundingMode=Floor  overflowMode=off  truncOrWrapMode=Truncate  wrap_flag=None
  Selector1 : Selector  NumberOfDimensions=2  IndexMode=Zero-based  InputPortWidth=3  IndexOptions=Select all,Index vector (port)  Indices=-1,0
  Selector3 : Selector  NumberOfDimensions=2  IndexMode=Zero-based  InputPortWidth=3  IndexOptions=Select all,Index vector (port)  Indices=-1,0
  Submatrix : dspmtrx3/Submatrix  RowSpan=Range of rows  RowStartMode=Index  RowStartIndex=41  RowEndMode=Last  RowEndIndex=1  ColSpan=All columns  ColStartMode=First  ColStartIndex=1  ColEndMode=Last  ColEndIndex=1
  Unit Delay External IC : simulink/Additional Math & Discrete/Additional Discrete/Unit Delay External IC  tsamp=-1
  Residual : Outport
  wires:
  For Iterator/1 -> Selector3/2, Compare To Constant2/1, Selector1/2, Decode Remaining Sub-Blocks (4.3 - 4.4)/5
  Frame Conversion1/1 -> Submatrix/1
  Selector3/1 -> Decode Remaining Sub-Blocks (4.3 - 4.4)/3
  Selector1/1 -> Decode Remaining Sub-Blocks (4.3 - 4.4)/4
  Unit Delay External IC/1 -> Frame Conversion3/1
  Gain Indices/1 -> Selector1/1
  Code Indices/1 -> Selector3/1
  Initial Codebook/1 -> Pad/1
  Decode Remaining Sub-Blocks (4.3 - 4.4)/1 -> Residual/1, Frame Conversion1/1
  Submatrix/1 -> Unit Delay External IC/1
  Pad/1 -> Unit Delay External IC/2
  Frame Conversion3/1 -> Decode Remaining Sub-Blocks (4.3 - 4.4)/1
  Compare To Constant2/1 -> Decode Remaining Sub-Blocks (4.3 - 4.4)/2
  Start State Number/1 -> Decode Remaining Sub-Blocks (4.3 - 4.4)/6
  State First/1 -> Decode Remaining Sub-Blocks (4.3 - 4.4)/7

== system dspilbc/iLBC Decoder/Decode Sub-Blocks (4.1 - 4.4)/Decoder LPC Analysis (4.1) ==
  LSF Indices : Inport
  Concatenation of Quantized LSFs : Concatenate  NumInputs=3  Mode=Multidimensional array
  Find Synthesis Filters (3.2.6) : dspilbclib/Find LPC Filters
  Frame Conversion1 : FrameConversion
  Selector3 : Selector  NumberOfDimensions=2  InputPortWidth=3  IndexOptions=Index vector (dialog),Select all  Indices=1,-1
  Selector4 : Selector  NumberOfDimensions=2  InputPortWidth=3  IndexOptions=Index vector (dialog),Select all  Indices=2,-1
  Selector5 : Selector  NumberOfDimensions=2  InputPortWidth=3  IndexOptions=Index vector (dialog),Select all  Indices=3,-1
  Sort : dspstat3/Sort  otype=Value  dir=Ascending  sortAlg=Quick sort  roundingMode=Floor  overflowMode=off
  Vector Quantizer Decoder1 : dspquant2/Vector Quantizer Decoder  invalidin=Clip  CBsource=Specify via dialog  codebook=ilbc.lsfCbTbl1  dataType=Inherit via back propagation  isSigned=on  wordLen=16  udDataType=float('single')  fracBitsMode=Best precision  numFracBits=7  OutDataTypeStr=Inherit: Inherit via back propagation  LastOutDataTypeStr=Inherit: Inherit via back propagation
  Vector Quantizer Decoder2 : dspquant2/Vector Quantizer Decoder  invalidin=Clip  CBsource=Specify via dialog  codebook=ilbc.lsfCbTbl2  dataType=Inherit via back propagation  isSigned=on  wordLen=16  udDataType=float('single')  fracBitsMode=Best precision  numFracBits=7  OutDataTypeStr=Inherit: Inherit via back propagation  LastOutDataTypeStr=Inherit: Inherit via back propagation
  Vector Quantizer Decoder3 : dspquant2/Vector Quantizer Decoder  invalidin=Clip  CBsource=Specify via dialog  codebook=ilbc.lsfCbTbl3  dataType=Inherit via back propagation  isSigned=on  wordLen=16  udDataType=float('single')  fracBitsMode=Best precision  numFracBits=7  OutDataTypeStr=Inherit: Inherit via back propagation  LastOutDataTypeStr=Inherit: Inherit via back propagation
  Synthesis : Outport
  wires:
  Frame Conversion1/1 -> Selector3/1, Selector4/1, Selector5/1
  Find Synthesis Filters (3.2.6)/1 -> Synthesis/1
  Sort/1 -> Find Synthesis Filters (3.2.6)/1
  Concatenation of Quantized LSFs/1 -> Sort/1
  Vector Quantizer Decoder3/1 -> Concatenation of Quantized LSFs/3
  Vector Quantizer Decoder2/1 -> Concatenation of Quantized LSFs/2
  Vector Quantizer Decoder1/1 -> Concatenation of Quantized LSFs/1
  LSF Indices/1 -> Frame Conversion1/1
  Selector5/1 -> Vector Quantizer Decoder3/1
  Selector4/1 -> Vector Quantizer Decoder2/1
  Selector3/1 -> Vector Quantizer Decoder1/1

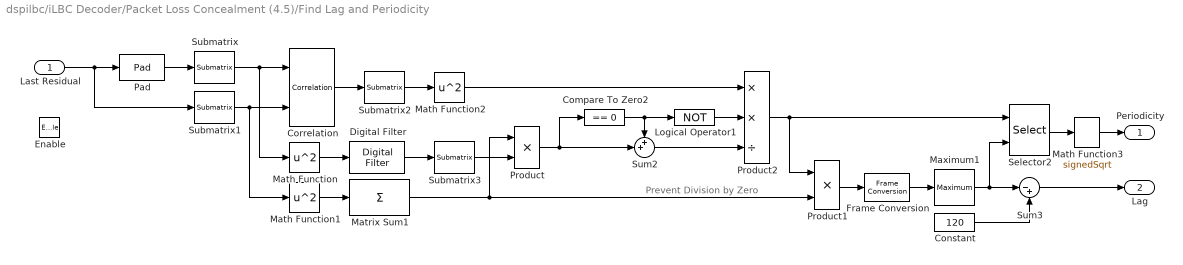
== system dspilbc/iLBC Decoder/Packet Loss Concealment (4.5)/Find Lag and Periodicity ==
  note: Prevent Division by Zero
  Last Residual : Inport
  Enable : EnablePort
  Compare To Zero2 : simulink/Logic and Bit Operations/Compare To Zero  relop===  OutDataTypeStr=uint8  ZeroCross=off
  Constant : Constant  Value=120  OutDataTypeStr=Inherit: Inherit via back propagation
  Correlation : dspstat3/Correlation  domain=Time  outputDataTypeStr=Inherit: Same as accumulator  outputLastDataTypeStr=Inherit: Same as accumulator  outputMin=[]  outputMax=[]  roundingMode=Floor  overflowMode=off
  Digital Filter : dsparch4/Digital Filter  TypePopup=FIR (all zeros)  IIRFiltStruct=Direct form II transposed  AllPoleFiltStruct=Direct form  FIRFiltStruct=Direct form  CoeffSource=Specify via dialog  NumCoeffs=ones(60,1)  DenCoeffs=[1 0.1]  BiQuadCoeffs=[1 0.3 0.4 1 0.1 0.2]  LatticeCoeffs=[0.2 0.4]  denIgnore=on  FiltPerSampPopup=One filter per frame  IC=0  ICnum=0  ICden=0  roundingMode=Floor  overflowMode=off  ScaleValues=1  scaleValueFracLength=14  stageInFracLength=15  stageOutFracLength=15  FilterSource=Specify via dialog  dfiltObjectName=dfilt.dffir([1 2 1])  InputProcessing=Columns as channels (frame based)
  Frame Conversion : FrameConversion  OutFrame=Sample-based
  Logical Operator1 : Logic  Operator=NOT  AllPortsSameDT=off  OutDataTypeStr=boolean
  Math Function : Math  Operator=square  SaturateOnIntegerOverflow=on
  Math Function1 : Math  Operator=square  SaturateOnIntegerOverflow=on
  Math Function2 : Math  Operator=square  SaturateOnIntegerOverflow=on
  Math Function3 : Sqrt  Operator=signedSqrt  AlgorithmType=Newton-Raphson  SaturateOnIntegerOverflow=on
  Matrix Sum1 : Sum  Inputs=+  CollapseMode=Specified dimension  OutDataTypeStr=Inherit: Same as accumulator
  Maximum1 : dspstat3/Maximum  fcn=Index  reset=None  InputProcessing=Columns as channels (frame based)  indexBase=Zero  operateOver=Each column  Dimension=1  colComp=on  operation=maximum  roiEnable=off  roiType=Rectangles  roiPortion=Entire ROI  roiOutput=Individual statistics for each ROI  roiFlag=off  accumDataTypeStr=Inherit: Same as product output  accumLastDataTypeStr=Inherit: Same as product output  roundingMode=Floor  overflowMode=off
  Pad : dspsigops/Pad  padAlong=Columns  dimsToPad=1  valSrc=Specify via dialog  padVal=0  spec=Output size  padNumOutRowsSpecMethod=User-specified  numOutRows=60+120  padNumOutColsSpecMethod=User-specified  numOutCols=1  isVarDimsMode=off  padBeginning=0  padEnd=0  outSizeMode=User-specified  outSize=1  padSigAt=Beginning  trunc_flag=None  roundingMode=Floor  overflowMode=off  truncOrWrapMode=Truncate  wrap_flag=None
  Product : Product  RndMeth=Zero
  Product1 : Product  RndMeth=Zero
  Product2 : Product  Inputs=**/  RndMeth=Zero
  Selector2 : Selector  NumberOfDimensions=2  IndexMode=Zero-based  InputPortWidth=3  IndexOptions=Index vector (port),Index vector (dialog)  Indices=[1 3],0  OutputSizes=7,1
  Submatrix : dspmtrx3/Submatrix  RowSpan=Range of rows  RowStartMode=First  RowStartIndex=120+60-1  RowEndMode=Offset from last  RowEndIndex=20  ColSpan=All columns  ColStartMode=First  ColStartIndex=1  ColEndMode=Last  ColEndIndex=1
  Submatrix1 : dspmtrx3/Submatrix  RowSpan=Range of rows  RowStartMode=Offset from last  RowStartIndex=60-1  RowEndMode=Last  RowEndIndex=60  ColSpan=All columns  ColStartMode=First  ColStartIndex=1  ColEndMode=Last  ColEndIndex=1
  Submatrix2 : dspmtrx3/Submatrix  RowSpan=Range of rows  RowStartMode=Index  RowStartIndex=60  RowEndMode=Offset from last  RowEndIndex=60-1  ColSpan=All columns  ColStartMode=First  ColStartIndex=1  ColEndMode=Last  ColEndIndex=1
  Submatrix3 : dspmtrx3/Submatrix  RowSpan=Range of rows  RowStartMode=Offset from last  RowStartIndex=100  RowEndMode=Last  RowEndIndex=101  ColSpan=All columns  ColStartMode=First  ColStartIndex=1  ColEndMode=Last  ColEndIndex=1
  Sum2 : Sum  Inputs=++|
  Sum3 : Sum  Inputs=|-+
  Periodicity : Outport
  Lag : Outport  Port=2
  wires:
  Compare To Zero2/1 -> Sum2/1, Logical Operator1/1
  Logical Operator1/1 -> Product2/2
  Submatrix3/1 -> Product/2
  Math Function3/1 -> Periodicity/1
  Constant/1 -> Sum3/2
  Frame Conversion/1 -> Maximum1/1
  Math Function2/1 -> Product2/1
  Maximum1/1 -> Sum3/1, Selector2/2
  Submatrix/1 -> Correlation/1, Math Function/1
  Submatrix1/1 -> Math Function1/1, Correlation/2
  Sum3/1 -> Lag/1
  Selector2/1 -> Math Function3/1
  Product2/1 -> Selector2/1, Product1/1
  Product1/1 -> Frame Conversion/1
  Sum2/1 -> Product2/3
  Product/1 -> Compare To Zero2/1, Sum2/2
  Matrix Sum1/1 -> Product/1, Product1/2
  Digital Filter/1 -> Submatrix3/1
  Math Function/1 -> Digital Filter/1
  Math Function1/1 -> Matrix Sum1/1
  Pad/1 -> Submatrix/1
  Submatrix2/1 -> Math Function2/1
  Correlation/1 -> Submatrix2/1
  Last Residual/1 -> Submatrix1/1, Pad/1

== system dspilbc/iLBC Decoder/Split Packet (3.8)/Unpack Packet ==
  Packet : Inport
  Assignment : Assignment  Indices=ilbc.bit_packTbl{ilbcMode}
  Bitwise Operator1 : simulink/Logic and Bit Operations/Bitwise Operator  logicop=AND  UseBitMask=on  BitMask=128  BitMaskRealWorld=Stored Integer
  Bitwise Operator2 : simulink/Logic and Bit Operations/Bitwise Operator  logicop=AND  UseBitMask=on  BitMask=64  BitMaskRealWorld=Stored Integer
  Bitwise Operator3 : simulink/Logic and Bit Operations/Bitwise Operator  logicop=AND  UseBitMask=on  BitMask=32  BitMaskRealWorld=Stored Integer
  Bitwise Operator4 : simulink/Logic and Bit Operations/Bitwise Operator  logicop=AND  UseBitMask=on  BitMask=16  BitMaskRealWorld=Stored Integer
  Bitwise Operator5 : simulink/Logic and Bit Operations/Bitwise Operator  logicop=AND  UseBitMask=on  BitMask=8  BitMaskRealWorld=Stored Integer
  Bitwise Operator6 : simulink/Logic and Bit Operations/Bitwise Operator  logicop=AND  UseBitMask=on  BitMask=4  BitMaskRealWorld=Stored Integer
  Bitwise Operator7 : simulink/Logic and Bit Operations/Bitwise Operator  logicop=AND  UseBitMask=on  BitMask=2  BitMaskRealWorld=Stored Integer
  Bitwise Operator8 : simulink/Logic and Bit Operations/Bitwise Operator  logicop=AND  UseBitMask=on  BitMask=1  BitMaskRealWorld=Stored Integer
  Compare To Constant : simulink/Logic and Bit Operations/Compare To Constant  relop=~=  const=0  OutDataTypeStr=boolean  ZeroCross=off
  Constant : Constant  Value=[128 64 32 16 8 4 2 1]'  VectorParams1D=off  OutDataTypeStr=uint8
  Matrix Concatenate : Concatenate  NumInputs=8  Mode=Multidimensional array
  Matrix Multiply : Product  Multiplication=Matrix(*)  OutDataTypeStr=uint8
  Reshape : Reshape  OutputDimensionality=Customize  OutputDimensions=[ilbc.UNPACKED_TBL_LEN{ilbcMode} 8]
  Zeros : Constant  Value=zeros(ilbc.UNPACKED_TBL_LEN{ilbcMode}*8,1)  VectorParams1D=off  OutDataTypeStr=boolean
  Values : Outport
  wires:
  Bitwise Operator8/1 -> Matrix Concatenate/8
  Bitwise Operator7/1 -> Matrix Concatenate/7
  Bitwise Operator6/1 -> Matrix Concatenate/6
  Bitwise Operator5/1 -> Matrix Concatenate/5
  Bitwise Operator4/1 -> Matrix Concatenate/4
  Bitwise Operator3/1 -> Matrix Concatenate/3
  Bitwise Operator2/1 -> Matrix Concatenate/2
  Bitwise Operator1/1 -> Matrix Concatenate/1
  Packet/1 -> Bitwise Operator3/1, Bitwise Operator4/1, Bitwise Operator5/1, Bitwise Operator6/1, Bitwise Operator7/1, Bitwise Operator8/1, Bitwise Operator2/1, Bitwise Operator1/1
  Matrix Multiply/1 -> Values/1
  Matrix Concatenate/1 -> Compare To Constant/1
  Constant/1 -> Matrix Multiply/2
  Reshape/1 -> Matrix Multiply/1
  Assignment/1 -> Reshape/1
  Compare To Constant/1 -> Assignment/2
  Zeros/1 -> Assignment/1
